simulink model "POHR_Stromregelung"  (R2021b)
settings: Solver=FixedStepAuto  StartTime=0.0  StopTime=stop_time  FixedStep=time_step  RelTol=1e-3
values from neighbouring files (symbols this model uses):
  BW = 1000    [PMSM_01_Parameter.m]    (also in POHR_Parameter.m = 800)
  L_max = 2*1.9957e-3    (= 0.0039914)    [POHR_Parameter.m]
  L_table = [L_max L_max L_min L_min L_max L_max]    [POHR_Parameter.m]
  n_speed = 3000    [POHR_Parameter.m]
  R = R_s    (= 0.079)    [CodeGenParams.m]    (also in PMSM_01_Parameter.m = 0.04; POHR_Parameter.m = 0.088)
  T_controller = 1/f_CurrentController    (= 0.0001)    [PMSM_01_Parameter.m]    (also in POHR_Parameter.m)
  theta_mech = [0 5 85 95 175 180] .* pi/180    [POHR_Parameter.m]
  time_step = T_controller/1000    (= 1e-07)    [POHR_Parameter.m]
undefined symbols (not defined in the file or in its folder): Ki, Kp
libraries: fl_lib x4, nesl_utility x4, embmathops x2, dspswit3 x2, ee_lib x1, slpidlib x1
settings Model: Creator=timow  LastModifiedBy=timow

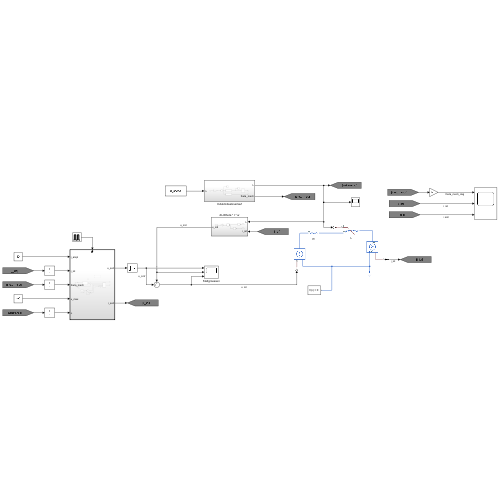
[thumbnail: Simulink's stored preview of the top-level diagram]
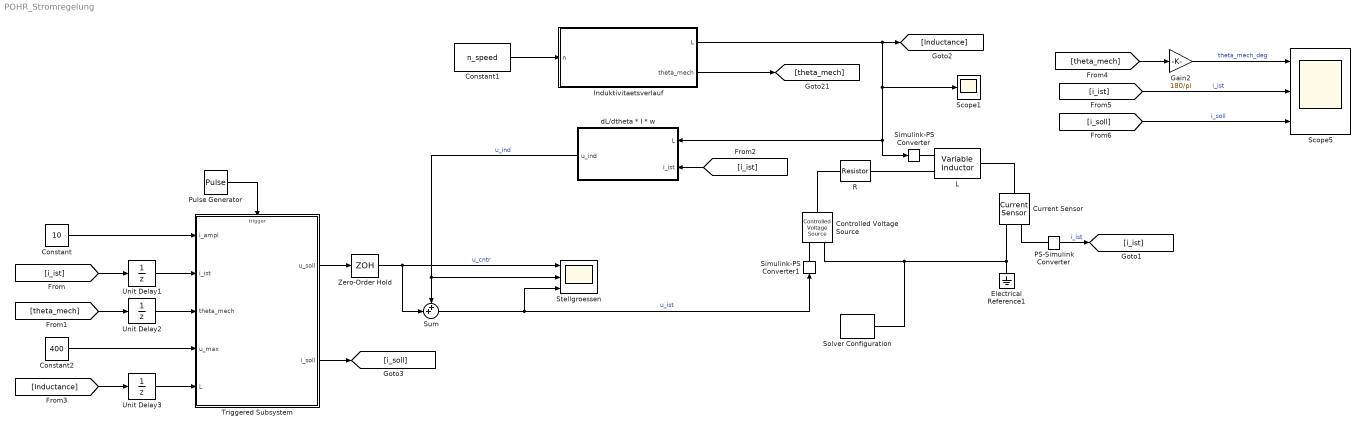
== system POHR_Stromregelung ==
  Constant : Constant  Value=10
  Constant1 : Constant  Value=n_speed
  Constant2 : Constant  Value=400
  Controlled Voltage Source : fl_lib/Electrical/Electrical Sources/Controlled Voltage Source
  Current Sensor : fl_lib/Electrical/Electrical Sensors/Current Sensor
  Electrical Reference1 : fl_lib/Electrical/Electrical Elements/Electrical Reference
  Gain2 : Gain  Gain=180/pi
  Induktivitaetsverlauf : Subsystem
  L : ee_lib/Passive/Variable Inductor  prm=1  Lmin=1e-6 H  g=1e-9 1/Ohm  i0=0 A  phi0=0 Wb
      settings: SourceProductBaseCode=PS  InternalSimscapePortConfiguration="{\"Bottom\":[],\"Left\":[{\"id\":\"L\",\"label\":\"L\",\"type\":\"input\"},{\"id\":\"p\",\"label\":\"+\",\"type\":\"foundation.electrical.electrical\"}],\"Right\":[{\"id\":\"n\",\"label\":\"-\",\"type\":\"foundation.electrical.electrical\"}],\"Top\":[]}"
  PS-Simulink Converter : nesl_utility/PS-Simulink Converter  PhysicalDomain=network_engine_domain  SubClassName=ps_output  LeftPortType=input  RightPortType=output  PseudoPeriodic=off  Frequencies=[]  Unit=inherit  AffineConversion=off
      settings: SourceProductBaseCode=PW,SS
  Pulse Generator : DiscretePulseGenerator  PulseType=Time based  Period=T_controller  PulseWidth=50
  R : fl_lib/Electrical/Electrical Elements/Resistor  R=R Ohm  i_specify=off  i_priority=None  i=0 A  i_nominal_specify=off  i_nominal_unit=A  i_nominal_value=1  v_specify=off  v_priority=None  v=0 V  v_nominal_specify=off  v_nominal_unit=V  v_nominal_value=1
  Scope1 : Scope
  Scope5 : Scope  NumInputPorts=3
  Simulink-PS Converter : nesl_utility/Simulink-PS Converter  PhysicalDomain=network_engine_domain  SubClassName=ps_input  LeftPortType=input  RightPortType=output  PseudoPeriodic=off  Frequencies=[]  NoiseDistribution=none  NoiseParameters=[]  Unit=1  AffineConversion=off  FilteringAndDerivatives=provide  SimscapeFilterOrder=1  InputFilterTimeConstant=0.001  UdotUserProvided=0
      settings: SourceProductBaseCode=PW,SS
  Simulink-PS Converter1 : nesl_utility/Simulink-PS Converter  PhysicalDomain=network_engine_domain  SubClassName=ps_input  LeftPortType=input  RightPortType=output  PseudoPeriodic=off  Frequencies=[]  NoiseDistribution=none  NoiseParameters=[]  Unit=1  AffineConversion=off  FilteringAndDerivatives=provide  SimscapeFilterOrder=1  InputFilterTimeConstant=0.001  UdotUserProvided=0
      settings: SourceProductBaseCode=PW,SS
  Solver Configuration : nesl_utility/Solver Configuration  PhysicalDomain=network_engine_domain  SubClassName=solver  LeftPortType=input  RightPortType=generic  Tones=[]  Harmonics=[]  SimulateNoise=off  Profile=off  UseLocalSampling=off  EnableSwitchedLinearOptims=on  FrequencyDomain=off  UseCCode=off  RelTol=0.001  AbsTol=1e-06  MinStep=1e-09  ToWorkspace=off  RevertToSquareIcSolve=off  NumHomotopyIterations=100  PhasorMode=off  PhasorModeNumHarmonics=1  DoDC=off  ResidualTolerance=1e-09  UseLocalSolver=off  LocalSolverChoice=NE_BACKWARD_EULER_ADVANCER  LocalSolverSampleTime=0.001  DoFixedCost=off  MaxNonlinIter=3  MaxModeIter=2  ComputeImpulses=off  ImpulseIterations=2  LinearAlgebra=auto  EquationFormulation=NE_TIME_EF  DelaysMemoryBudget=1024  AutomaticFiltering=on  FilteringTimeConstant=0.001  PartitionStorageMethod=AS_NEEDED  PartitionMemoryBudget=1024  PartitionMethod=ROBUST
      settings: SourceProductBaseCode=PW,SS
  Stellgroessen : Scope  NumInputPorts=3
  Sum : Sum  Inputs=++|
  Triggered Subsystem : Subsystem  TreatAsAtomicUnit=on
  Unit Delay1 : UnitDelay  SampleTime=time_step  HasFrameUpgradeWarning=on
  Unit Delay2 : UnitDelay  SampleTime=time_step  HasFrameUpgradeWarning=on
  Unit Delay3 : UnitDelay  SampleTime=time_step  HasFrameUpgradeWarning=on
  Zero-Order Hold : ZeroOrderHold  SampleTime=T_controller
  dL/dtheta * I * w : Subsystem
  wires:
  PS-Simulink Converter/1 -> [i_ist]  "i_ist"
  Pulse Generator/1 -> Triggered Subsystem/Trigger
  Constant/1 -> Triggered Subsystem/1(i_ampl)
  Unit Delay1/1 -> Triggered Subsystem/2(i_ist)
  [i_ist] -> Unit Delay1/1
  Unit Delay2/1 -> Triggered Subsystem/3(theta_mech)
  [theta_mech] -> Unit Delay2/1
  Constant2/1 -> Triggered Subsystem/4(u_max)
  Zero-Order Hold/1 -> Stellgroessen/1, Sum/2  "u_cntr"
  Sum/1 -> Stellgroessen/3, Simulink-PS Converter1/1  "u_ist"
  Triggered Subsystem/1(u_soll) -> Zero-Order Hold/1
  [Inductance] -> Unit Delay3/1
  Unit Delay3/1 -> Triggered Subsystem/5(L)
  [theta_mech] -> Gain2/1
  [i_ist] -> Scope5/2  "i_ist"
  Gain2/1 -> Scope5/1  "theta_mech_deg"
  Induktivitaetsverlauf/1(L) -> Simulink-PS Converter/1, dL/dtheta * I * w/1(L), Scope1/1, [Inductance]
  Constant1/1 -> Induktivitaetsverlauf/1(n)
  dL/dtheta * I * w/1(u_ind) -> Stellgroessen/2, Sum/1  "u_ind"
  Triggered Subsystem/2(i_soll) -> [i_soll]
  [i_soll] -> Scope5/3  "i_soll"
  Induktivitaetsverlauf/2(theta_mech) -> [theta_mech]
  [i_ist] -> dL/dtheta * I * w/2(i_ist)
  connections:
  R/RConn1 -- L/LConn2
  Controlled Voltage Source/LConn1 -- R/LConn1
  Electrical Reference1/LConn1 -- Current Sensor/RConn2 -- Solver Configuration/RConn1 -- Controlled Voltage Source/RConn2
  Simulink-PS Converter/RConn1 -- L/LConn1
  Simulink-PS Converter1/RConn1 -- Controlled Voltage Source/RConn1
  L/RConn1 -- Current Sensor/LConn1
  Current Sensor/RConn1 -- PS-Simulink Converter/LConn1

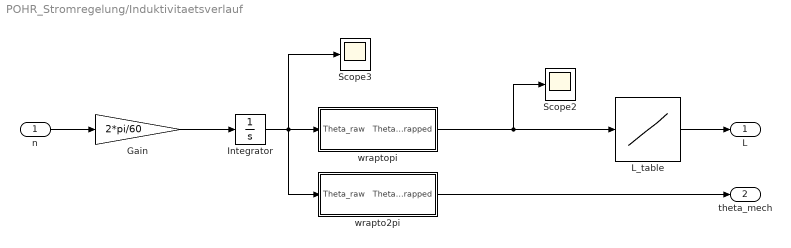
== system POHR_Stromregelung/Induktivitaetsverlauf ==
  n : Inport
  Gain : Gain  Gain=2*pi/60
  Integrator : Integrator  WrappedStateUpperValue=pi/2  WrappedStateLowerValue=0
  L_table : Lookup_n-D  NumberOfTableDimensions=1  BreakpointsForDimension1=theta_mech  Table=L_table  InternalRulePriority=Speed  RndMeth=Simplest  InputSameDT=on
  Scope2 : Scope
  Scope3 : Scope
  wrapto2pi : Subsystem
  wraptopi : Subsystem
  L : Outport
  theta_mech : Outport  Port=2
  wires:
  wraptopi/1(Theta_wrapped) -> L_table/1, Scope2/1
  Integrator/1 -> wrapto2pi/1(Theta_raw), wraptopi/1(Theta_raw), Scope3/1
  n/1 -> Gain/1
  Gain/1 -> Integrator/1
  L_table/1 -> L/1
  wrapto2pi/1(Theta_wrapped) -> theta_mech/1

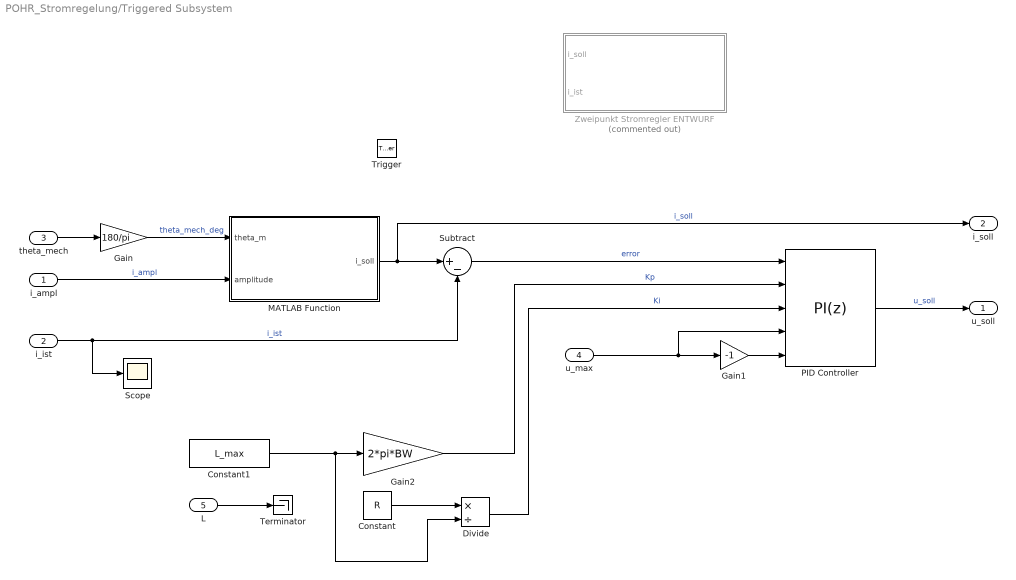
== system POHR_Stromregelung/Triggered Subsystem ==
  i_ampl : Inport
  i_ist : Inport  Port=2
  theta_mech : Inport  Port=3
  u_max : Inport  Port=4
  L : Inport  Port=5
  Trigger : TriggerPort  VariantControl=(inherit)
  Constant : Constant  Value=R
  Constant1 : Constant  Value=L_max
  Divide : Product  Inputs=*/
  Gain : Gain  Gain=180/pi
  Gain1 : Gain  Gain=-1
  Gain2 : Gain  Gain=2*pi*BW
  MATLAB Function : MATLAB Function  TreatAsAtomicUnit=on
  PID Controller : slpidlib/PID Controller  Controller=PI  Form=Parallel  TimeDomain=Discrete-time  UseExternalTs=off  SampleTime=-1  IntegratorMethod=Forward Euler  FilterMethod=Forward Euler  ControllerParametersSource=external  P=Kp  I=Ki  D=0  UseFilter=on  N=100  TunerSelectOption=Transfer Function Based (PID Tuner App)  InitialConditionSource=internal  InitialConditionForIntegrator=0  InitialConditionForFilter=0  DifferentiatorICPrevScaledInput=0  ExternalReset=none  TrackingMode=off  Kt=1  LimitOutput=on  SatLimitsSource=external  UpperSaturationLimit=inf  LowerSaturationLimit=-inf  LinearizeAsGain=on  AntiWindupMode=clamping  Kb=1  POutMin=[]  POutMax=[]  IOutMin=[]  IOutMax=[]  DOutMin=[]  DOutMax=[]  NOutMin=[]  NOutMax=[]  SumOutMin=[]  SumOutMax=[]  SaturationOutMin=[]  SaturationOutMax=[]  PParamMin=[]  PParamMax=[]  IParamMin=[]  IParamMax=[]  DParamMin=[]  DParamMax=[]  NParamMin=[]  NParamMax=[]  KbParamMin=[]  KbParamMax=[]  KtParamMin=[]  KtParamMax=[]  KbOutMin=[]  KbOutMax=[]  KtOutMin=[]  KtOutMax=[]  IntegratorOutMin=[]  IntegratorOutMax=[]  FilterOutMin=[]  FilterOutMax=[]  SumI1OutMin=[]  SumI1OutMax=[]  SumI2OutMin=[]  SumI2OutMax=[]  SumI3OutMin=[]  SumI3OutMax=[]  SumI4OutMin=[]  SumI4OutMax=[]  SumDOutMin=[]  SumDOutMax=[]  DifferentiatorOutMin=[]  DifferentiatorOutMax=[]  FilterDiffOutCoefMin=[]  FilterDiffOutCoefMax=[]  ReciprocalOutMin=[]  ReciprocalOutMax=[]  SumDenOutMin=[]  SumDenOutMax=[]  SumNumOutMin=[]  SumNumOutMax=[]  DivideOutMin=[]  DivideOutMax=[]  UdiffTsProdOutMin=[]  UdiffTsProdOutMax=[]  NTsProdOutMin=[]  NTsProdOutMax=[]  UintegralTsProdOutMin=[]  UintegralTsProdOutMax=[]  UngainTsProdOutMin=[]  UngainTsProdOutMax=[]  IntegratorContinuousStateAttributes=''  IntegratorStateMustResolveToSignalObject=off  IntegratorRTWStateStorageClass=Auto  FilterContinuousStateAttributes=''  FilterStateMustResolveToSignalObject=off  FilterRTWStateStorageClass=Auto  ParallelPVariant=ExternalParameters  IdealPVariant=Disabled  IVariant=ExternalParameters  DVariant=Disabled  IntegratorVariant=Discrete  SatVariant=External  AWVariant=DiscClampingParallel  PCopyVariant=Disabled  TRVariant=Disabled  FdbkBlocksVariant=Forward  IdealPFdbkVariant=Disabled  SatFdbkVariant=Disabled  DerivativeFilterVariant=Disabled  NVariant=Disabled  NCopyVariant=Disabled_SignalSpec  FilterICVariant=Disabled  IntegratorICVariant=InternalICs  ExternalResetVariant=Disabled  TRSumVariant=Passthrough  SumFdbkVariant=Disabled  SumVariant=Sum_PI  TsampFilterVariant=InternalTs  TsampNgainVariant=Passthrough  TsampIntegralVariant=Passthrough  ExternalSaturationOutDataTypeStr=Inherit: Same as second input
  Scope : Scope
  Subtract : Sum  Inputs=|+-
  Terminator : Terminator
  Zweipunkt Stromregler ENTWURF : Subsystem  Commented=on
  u_soll : Outport
  i_soll : Outport  Port=2
  wires:
  Subtract/1 -> PID Controller/1  "error"
  i_ampl/1 -> MATLAB Function/2(amplitude)  "i_ampl"
  Gain/1 -> MATLAB Function/1(theta_m)  "theta_mech_deg"
  theta_mech/1 -> Gain/1
  i_ist/1 -> Scope/1, Subtract/2  "i_ist"
  PID Controller/1 -> u_soll/1  "u_soll"
  u_max/1 -> PID Controller/4, Gain1/1
  Gain1/1 -> PID Controller/5
  Constant/1 -> Divide/1
  Constant1/1 -> Gain2/1, Divide/2
  Gain2/1 -> PID Controller/2  "Kp"
  Divide/1 -> PID Controller/3  "Ki"
  L/1 -> Terminator/1
  MATLAB Function/1(i_soll) -> i_soll/1, Subtract/1  "i_soll"

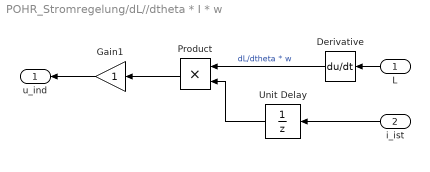
== system POHR_Stromregelung/dL//dtheta * I * w ==
  L : Inport
  i_ist : Inport  Port=2
  Derivative : Derivative
  Gain1 : Gain
  Product : Product
  Unit Delay : UnitDelay  SampleTime=time_step  HasFrameUpgradeWarning=on
  u_ind : Outport
  wires:
  Product/1 -> Gain1/1
  Derivative/1 -> Product/1  "dL/dtheta * w"
  i_ist/1 -> Unit Delay/1
  Unit Delay/1 -> Product/2
  L/1 -> Derivative/1
  Gain1/1 -> u_ind/1

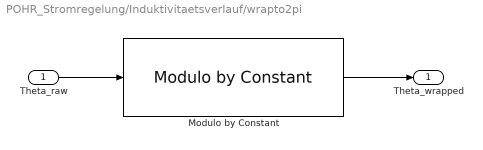
== system POHR_Stromregelung/Induktivitaetsverlauf/wrapto2pi ==
  Theta_raw : Inport
  Modulo by Constant : embmathops/Modulo by Constant  Denominator=2*pi  SimulateUsing=Code generation
      settings: SourceProductBaseCode=SL
  Theta_wrapped : Outport
  wires:
  Theta_raw/1 -> Modulo by Constant/1
  Modulo by Constant/1 -> Theta_wrapped/1

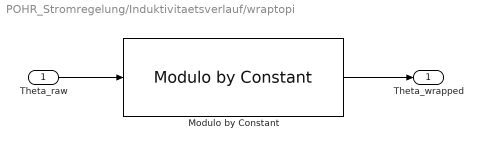
== system POHR_Stromregelung/Induktivitaetsverlauf/wraptopi ==
  Theta_raw : Inport
  Modulo by Constant : embmathops/Modulo by Constant  Denominator=pi  SimulateUsing=Code generation
      settings: SourceProductBaseCode=SL
  Theta_wrapped : Outport
  wires:
  Theta_raw/1 -> Modulo by Constant/1
  Modulo by Constant/1 -> Theta_wrapped/1

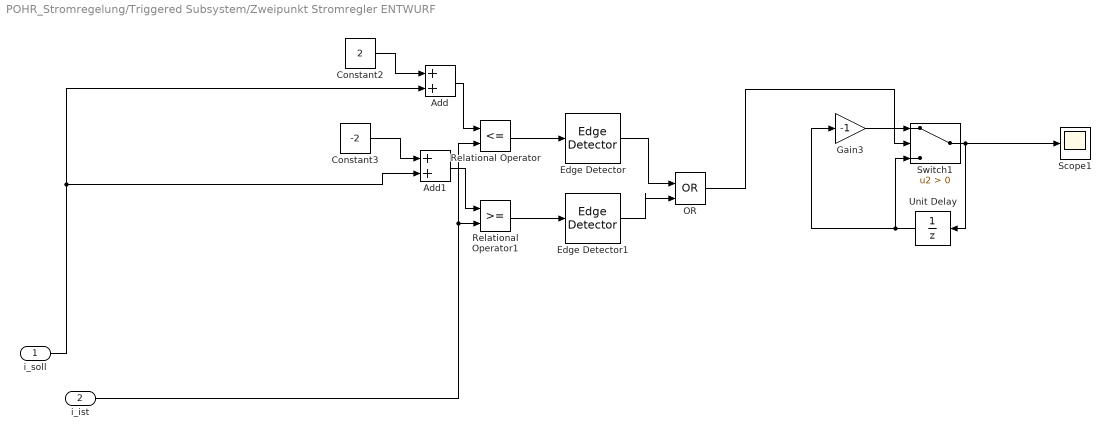
== system POHR_Stromregelung/Triggered Subsystem/Zweipunkt Stromregler ENTWURF ==
  i_soll : Inport
  i_ist : Inport  Port=2
  Add : Sum
  Add1 : Sum
  Constant2 : Constant  Value=2
  Constant3 : Constant  Value=-2
  Edge Detector : dspswit3/Edge Detector  InputProcessing=Columns as channels (frame based)
      settings: SourceProductBaseCode=DS
  Edge Detector1 : dspswit3/Edge Detector  InputProcessing=Columns as channels (frame based)
      settings: SourceProductBaseCode=DS
  Gain3 : Gain  Gain=-1
  OR : Logic  Operator=OR  IconShape=distinctive  AllPortsSameDT=off  OutDataTypeStr=boolean
  Relational Operator : RelationalOperator  Operator=<=  OutDataTypeStr=boolean  RndMeth=Simplest
  Relational Operator1 : RelationalOperator  OutDataTypeStr=boolean  RndMeth=Simplest
  Scope1 : Scope
  Switch1 : Switch  Criteria=u2 > Threshold
  Unit Delay : UnitDelay  InitialCondition=-100  SampleTime=-1  HasFrameUpgradeWarning=on
  wires:
  i_soll/1 -> Add1/2, Add/2
  Add/1 -> Relational Operator/1
  Relational Operator1/1 -> Edge Detector1/1
  Unit Delay/1 -> Gain3/1, Switch1/3
  Constant2/1 -> Add/1
  Switch1/1 -> Scope1/1, Unit Delay/1
  Gain3/1 -> Switch1/1
  Add1/1 -> Relational Operator1/1
  Constant3/1 -> Add1/1
  i_ist/1 -> Relational Operator/2, Relational Operator1/2
  Edge Detector1/1 -> OR/2
  OR/1 -> Switch1/2
  Edge Detector/1 -> OR/1
  Relational Operator/1 -> Edge Detector/1

== matlab function POHR_Stromregelung/Triggered Subsystem/MATLAB Function ==
  data: theta_m input; i_soll output; amplitude input
function i_soll = fcn(theta_m, amplitude)


if (theta_m >= 120 && theta_m <= 175) || (theta_m >= 300 && theta_m <= 355)
    i_val = amplitude;
else
    i_val = 0.0;
end

i_soll = i_val;
